simulink subsystem "ForwardFusionTrackerMetrics"  (R2022a)
settings: Solver=VariableStepAuto  StartTime=0.0  StopTime=10.0  RelTol=1e-3
libraries: simulink x4, trackmetricslib x1
settings Model: Creator=The MathWorks, Inc.  LastModifiedBy=The MathWorks, Inc.
settings SolverCC: MaxZcPerStep=1
settings DebuggingCC: UnconnectedInputMsg=warning  UnconnectedOutputMsg=warning  UnconnectedLineMsg=warning
settings RTWCC: DLArmComputeVersion=19.05

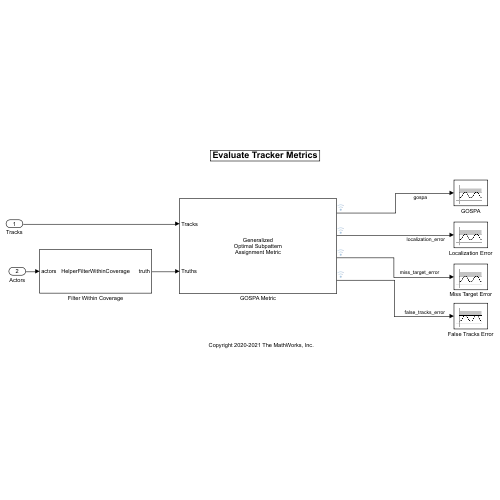
[thumbnail: Simulink's stored preview of the top-level diagram]
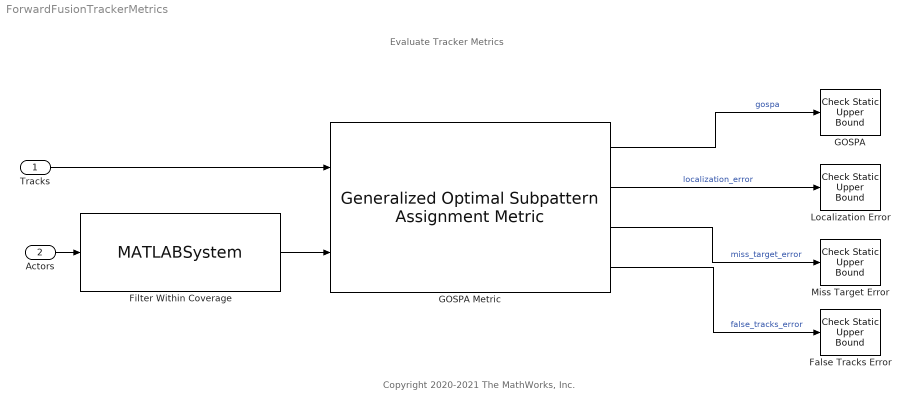
== system ForwardFusionTrackerMetrics ==
  note: Evaluate Tracker Metrics
  note: Copyright 2020-2021 The MathWorks, Inc.
  Tracks : Inport
  Actors : Inport  Port=2
  False Tracks Error : simulink/Model Verification/Check Static  Upper Bound  Description=u <= assessment.FalseTracksError  max=assessment.FalseTracksError  max_included=on  enabled=on  stopWhenAssertionFail=off  export=off  icon=graphic
      settings: SourceProductBaseCode=SL
  Filter Within Coverage : MATLABSystem  System=HelperFilterWithinCoverage  Camera=camera  Radar=radar  OutputBusName=BusSimulation3DActors1
      mask Type: HelperFilterWithinCoverage
      mask Display:
      | disp('HelperFilterWithinCoverage');
      | port_label('input',1,'actors');
      | port_label('output',1,'truth');
  GOSPA : simulink/Model Verification/Check Static  Upper Bound  Description=u <= assessment.GOSPA  max=assessment.GOSPA  max_included=on  enabled=on  stopWhenAssertionFail=off  export=off  icon=graphic
      settings: SourceProductBaseCode=SL
  GOSPA Metric : trackmetricslib/Generalized Optimal Subpattern Assignment Metric  CutoffDistance=cutOffDistance  Order=order  Alpha=alpha  Distance=custom  MotionModel=constvel  DistanceFcn=helperComputeDistanceToTruth  SwitchingPenalty=switchingPenalty  SimulateUsing=Interpreted execution  HasAssignmentInput=off  EnableGOSPAOutput=off  EnableSwitchingGOSPAOutput=off  EnableLocalizationGOSPAOutput=on  EnableMissedTargetGOSPAOutput=on  EnableFalseTrackGOSPAOutput=on  TrackFormat=objectTrack  TruthFormat=Actor
      settings: SourceProductBaseCode=TF
  Localization Error : simulink/Model Verification/Check Static  Upper Bound  Description=u <= assessment.LocalizationError  max=assessment.LocalizationError  max_included=on  enabled=on  stopWhenAssertionFail=off  export=off  icon=graphic
      settings: SourceProductBaseCode=SL
  Miss Target Error : simulink/Model Verification/Check Static  Upper Bound  Description=u <= assessment.MissTargetError  max=assessment.MissTargetError  max_included=on  enabled=on  stopWhenAssertionFail=off  export=off  icon=graphic
      settings: SourceProductBaseCode=SL
  wires:
  Actors/1 -> Filter Within Coverage/1
  Tracks/1 -> GOSPA Metric/1
  GOSPA Metric/1 -> GOSPA/1  "gospa"
  GOSPA Metric/2 -> Localization Error/1  "localization_error"
  GOSPA Metric/3 -> Miss Target Error/1  "miss_target_error"
  GOSPA Metric/4 -> False Tracks Error/1  "false_tracks_error"
  Filter Within Coverage/1 -> GOSPA Metric/2
